simulink model "practice7"  (Simulink 7.9)
settings: Solver=ode45  StartTime=0.0  StopTime=6  RelTol=1e-3
settings Model: Creator=sony  LastModifiedBy=sony

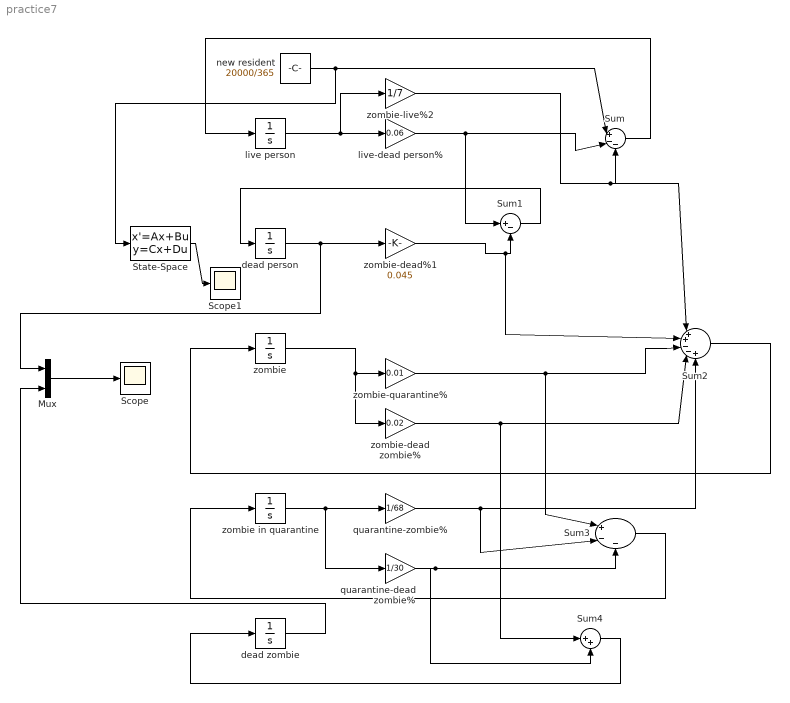
== system practice7 ==
  Mux : Mux  Inputs=2
  Scope : Scope
  Scope1 : Scope
  State-Space : StateSpace  A=[-(1/7+0.06) 0 0 0 0;0.06 -0.045 0 0 0;1/7 0.045 -0.03 1/68 0;0 0 0.01 -(1/68+1/30) 0;0 0 0.02 1/30 0]  B=[1;0;0;0;0]  C=[0 1 0 0 0;0 0 0 0 1]  D=[0;0]  X0=[300000;0;1;0;0]
  Sum : Sum  Inputs=|+--
  Sum1 : Sum  Inputs=|+-
  Sum2 : Sum  Inputs=|++--+
  Sum3 : Sum  Inputs=|+--
  Sum4 : Sum  Inputs=|++
  dead person : Integrator
  dead zombie : Integrator
  live person : Integrator  InitialCondition=300000
  live-dead person% : Gain  Gain=0.06
  new resident : Constant  Value=20000/365
  quarantine-dead zombie% : Gain  Gain=1/30
  quarantine-zombie% : Gain  Gain=1/68
  zombie : Integrator  InitialCondition=1
  zombie in quarantine : Integrator
  zombie-dead zombie% : Gain  Gain=0.02
  zombie-dead%1 : Gain  Gain=0.045
  zombie-live%2 : Gain  Gain=1/7
  zombie-quarantine% : Gain  Gain=0.01
  wires:
  new resident/1 -> Sum/1, State-Space/1
  live person/1 -> live-dead person%/1, zombie-live%2/1
  zombie/1 -> zombie-dead zombie%/1, zombie-quarantine%/1
  live-dead person%/1 -> Sum/2, Sum1/1
  Sum/1 -> live person/1
  Sum1/1 -> dead person/1
  zombie in quarantine/1 -> quarantine-zombie%/1, quarantine-dead zombie%/1
  quarantine-zombie%/1 -> Sum2/5, Sum3/2
  zombie-quarantine%/1 -> Sum2/3, Sum3/1
  zombie-dead zombie%/1 -> Sum2/4, Sum4/1
  Sum2/1 -> zombie/1
  quarantine-dead zombie%/1 -> Sum3/3, Sum4/2
  Sum3/1 -> zombie in quarantine/1
  Sum4/1 -> dead zombie/1
  Mux/1 -> Scope/1
  dead person/1 -> Mux/1, zombie-dead%1/1
  dead zombie/1 -> Mux/2
  zombie-live%2/1 -> Sum/3, Sum2/1
  zombie-dead%1/1 -> Sum1/2, Sum2/2
  State-Space/1 -> Scope1/1
